simulink model "quadcopter_plant_model"  (R2016b)
settings: Solver=VariableStepAuto  StartTime=0.0  StopTime=10.0  RelTol=1e-3
settings Model: Creator=aaronniemiec  LastModifiedBy=aaronniemiec

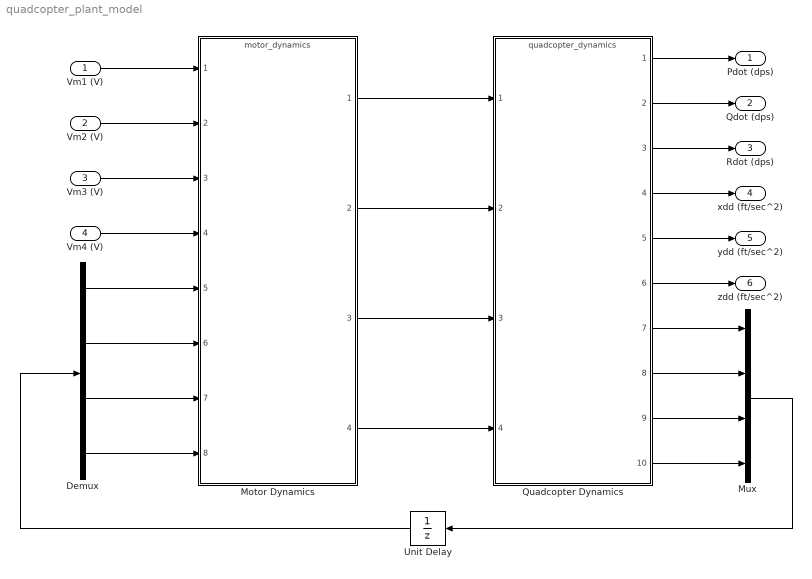
== system quadcopter_plant_model ==
  Vm1 (V) : Inport
  Vm2 (V) : Inport  Port=2
  Vm3 (V) : Inport  Port=3
  Vm4 (V) : Inport  Port=4
  Demux : Demux
  Motor Dynamics : ModelReference  ModelNameDialog=motor_dynamics.slx  SimulationMode=Normal  ModelReferenceVersion=1.2
  Mux : Mux
  Quadcopter Dynamics : ModelReference  ModelNameDialog=quadcopter_dynamics.slx  SimulationMode=Normal  ModelReferenceVersion=1.1
  Unit Delay : UnitDelay  SampleTime=-1
  Pdot (dps) : Outport
  Qdot (dps) : Outport  Port=2
  Rdot (dps) : Outport  Port=3
  xdd (ft/sec^2) : Outport  Port=4
  ydd (ft/sec^2) : Outport  Port=5
  zdd (ft/sec^2) : Outport  Port=6
  wires:
  Motor Dynamics/1 -> Quadcopter Dynamics/1
  Motor Dynamics/2 -> Quadcopter Dynamics/2
  Motor Dynamics/3 -> Quadcopter Dynamics/3
  Motor Dynamics/4 -> Quadcopter Dynamics/4
  Quadcopter Dynamics/7 -> Mux/1
  Quadcopter Dynamics/8 -> Mux/2
  Quadcopter Dynamics/9 -> Mux/3
  Quadcopter Dynamics/10 -> Mux/4
  Mux/1 -> Unit Delay/1
  Quadcopter Dynamics/1 -> Pdot (dps)/1
  Quadcopter Dynamics/2 -> Qdot (dps)/1
  Quadcopter Dynamics/3 -> Rdot (dps)/1
  Quadcopter Dynamics/4 -> xdd (ft/sec^2)/1
  Quadcopter Dynamics/5 -> ydd (ft/sec^2)/1
  Quadcopter Dynamics/6 -> zdd (ft/sec^2)/1
  Unit Delay/1 -> Demux/1
  Vm4 (V)/1 -> Motor Dynamics/4
  Vm3 (V)/1 -> Motor Dynamics/3
  Vm1 (V)/1 -> Motor Dynamics/1
  Vm2 (V)/1 -> Motor Dynamics/2
  Demux/3 -> Motor Dynamics/7
  Demux/4 -> Motor Dynamics/8
  Demux/1 -> Motor Dynamics/5
  Demux/2 -> Motor Dynamics/6
